simulink model "nms_3Dmodel_inv_wAnkleCPG"  (R2016b)
settings: Solver=ode3  StartTime=0.0  StopTime=tend  FixedStep=ts  RelTol=1e-3  EnableMultiTasking=on
InitFcn:
  | runScripts_inv;
values from neighbouring files (symbols this model uses):
  c = 0.05    [IID_nms_MechInit.m]    (also in nms_MechInit.m)
  c_jointstop = 0.3 / (pi/180)    (= 17.1887338539)    [IID_nms_MechInit.m]    (also in nms_MechInit.m)
  CPG_On = 1    [setCPGPar.m]    (also in setCPGPar_inv.m)
  CtrlPar_FP = [alpha0 alpha_cd alpha_cv]    [setCtrlPar.m]
  CtrlPar_FP_R = [R_hipR0 R_hipR_cd R_hipR_cv]    [setCtrlPar.m]
  CtrlPar_LL = l_clr    [setCtrlPar.m]
  CtrlPar_St = [StPreStim St_M1 St_M2 St_M3 St_M4 St_M5 St_M11]    [setCtrlPar.m]
  CtrlPar_St_R = [R_StPreStim R_St_M1 R_St_M3 R_St_M4]    [setCtrlPar.m]
  CtrlPar_Sw = [SwPreStim SwPhasePari SwPhaseParii SwCtrlPar_H SwCtrlPar_A      SwCtrlPar_Ki SwCtrlPar_Kii SwCtrlPar_Kiii SwCtrlPar_StP]    [setCtrlPar.m]
  CtrlPar_Sw_R = [R_SwPreStim R_Sw_M6]    [setCtrlPar.m]
  CtrlPar_theta0 = parBlCtrl(1)      *1*pi/180    [setCtrlPar.m]
  CtrlPar_Tr = [Tr_St_sup Tr_Sw]    [setCtrlPar.m]
  CtrlPar_Tr_R = [R_Tr_St_sup R_Tr_Sw]    [setCtrlPar.m]
  eref = 0.04    [IID_nms_MechInit.m]    (also in nms_MechInit.m)
  FmaxBFSH = 350    [nms_MechInit.m]
  FmaxGAS = 1500    [IID_nms_MechInit.m]    (also in nms_MechInit.m)
  FmaxGLU = 1500    [IID_nms_MechInit.m]    (also in nms_MechInit.m)
  FmaxHAB = 3000    [nms_MechInit.m]
  FmaxHAD = 4500    [nms_MechInit.m]
  FmaxHAM = 3000    [IID_nms_MechInit.m]    (also in nms_MechInit.m)
  FmaxHFL = 2000    [IID_nms_MechInit.m]    (also in nms_MechInit.m)
  FmaxRF = 1200    [nms_MechInit.m]
  FmaxSOL = 4000    [IID_nms_MechInit.m]    (also in nms_MechInit.m)
  FmaxTA = 800    [IID_nms_MechInit.m]    (also in nms_MechInit.m)
  FmaxVAS = 6000    [IID_nms_MechInit.m]    (also in nms_MechInit.m)
  init_a_tgt = 70*pi/180    (= 1.2217304764)    [setInitPar.m]
  init_a_tgtR = 90*pi/180    (= 1.57079632679)    [setInitPar.m]
  K = 5    [IID_nms_MechInit.m]    (also in nms_MechInit.m)
  leg_l = [D12_T D12_S]    [nms_MechInit.m]
  LongDelay = 0.020    (= 0.02)    [IID_setCtrlPar.m]    (also in nms_MechInit.m = 0.01)
  LongLoopDelay = 0.030    (= 0.03)    [nms_MechInit.m]
  loptBFSH = 0.12    [nms_MechInit.m]
  loptGAS = 0.05    [IID_nms_MechInit.m]    (also in nms_MechInit.m)
  loptGLU = 0.11    [IID_nms_MechInit.m]    (also in nms_MechInit.m)
  loptHAB = 0.09    [nms_MechInit.m]
  loptHAD = 0.10    (= 0.1)    [nms_MechInit.m]
  loptHAM = 0.10    (= 0.1)    [IID_nms_MechInit.m]    (also in nms_MechInit.m)
  loptHFL = 0.11    [IID_nms_MechInit.m]    (also in nms_MechInit.m)
  loptRF = 0.08    [nms_MechInit.m]
  loptSOL = 0.04    [IID_nms_MechInit.m]    (also in nms_MechInit.m)
  loptTA = 0.06    [IID_nms_MechInit.m]    (also in nms_MechInit.m)
  loptVAS = 0.08    [IID_nms_MechInit.m]    (also in nms_MechInit.m)
  lslackBFSH = 0.10    (= 0.1)    [nms_MechInit.m]
  lslackGAS = 0.40    (= 0.4)    [IID_nms_MechInit.m]    (also in nms_MechInit.m)
  lslackGLU = 0.13    [IID_nms_MechInit.m]    (also in nms_MechInit.m)
  lslackHAB = 0.07    [nms_MechInit.m]
  lslackHAD = 0.18    [nms_MechInit.m]
  lslackHAM = 0.31    [IID_nms_MechInit.m]    (also in nms_MechInit.m)
  lslackHFL = 0.10    (= 0.1)    [IID_nms_MechInit.m]    (also in nms_MechInit.m)
  lslackRF = 0.35    [nms_MechInit.m]
  lslackSOL = 0.26    [IID_nms_MechInit.m]    (also in nms_MechInit.m)
  lslackTA = 0.24    [IID_nms_MechInit.m]    (also in nms_MechInit.m)
  lslackVAS = 0.23    [IID_nms_MechInit.m]    (also in nms_MechInit.m)
  massBFSH = 2    [nms_MechInit.m]
  massGAS = 0.45    [IID_nms_MechInit.m]    (also in nms_MechInit.m)
  massGLU = 1.4    [IID_nms_MechInit.m]    (also in nms_MechInit.m)
  massHAB = 1.145    [nms_MechInit.m]
  massHAD = 1.91    [nms_MechInit.m]
  massHAM = 1.82    [IID_nms_MechInit.m]    (also in nms_MechInit.m)
  massHFL = 1.87    [IID_nms_MechInit.m]    (also in nms_MechInit.m)
  massRF = 1    [nms_MechInit.m]
  massSOL = 1.36    [IID_nms_MechInit.m]    (also in nms_MechInit.m)
  massTA = 0.29    [IID_nms_MechInit.m]    (also in nms_MechInit.m)
  massVAS = 2.91    [IID_nms_MechInit.m]    (also in nms_MechInit.m)
  MidDelay = 0.010    (= 0.01)    [IID_setCtrlPar.m]    (also in nms_MechInit.m = 0.005)
  N = 1.5    [IID_nms_MechInit.m]    (also in cmaes_parfor.m = size(x,1); nms_MechInit.m)
  phi12_LowLimit = 70*pi/180    (= 1.2217304764)    [IID_nms_MechInit.m]    (also in nms_MechInit.m)
  phi12_UpLimit = 130*pi/180    (= 2.26892802759)    [IID_nms_MechInit.m]    (also in nms_MechInit.m)
  phi23_UpLimit = 175*pi/180    (= 3.05432619099)    [IID_nms_MechInit.m]    (also in nms_MechInit.m)
  phi34_UpLimit = 230*pi/180    (= 4.01425727959)    [IID_nms_MechInit.m]    (also in nms_MechInit.m)
  phi34R_LowLimit = -15*pi/180    (= -0.261799387799)    [nms_MechInit.m]
  phi34R_UpLimit = 50*pi/180    (= 0.872664625997)    [nms_MechInit.m]
  phimaxGASa = 110*pi/180    (= 1.91986217719)    [IID_nms_MechInit.m]    (also in nms_MechInit.m = 1.74532925199)
  phimaxGASk = 140*pi/180    (= 2.44346095279)    [IID_nms_MechInit.m]    (also in nms_MechInit.m)
  phimaxRFk = 165*pi/180    (= 2.87979326579)    [nms_MechInit.m]
  phimaxSOL = 110*pi/180    (= 1.91986217719)    [IID_nms_MechInit.m]    (also in nms_MechInit.m = 1.74532925199)
  phimaxTA = 80*pi/180    (= 1.3962634016)    [IID_nms_MechInit.m]    (also in nms_MechInit.m)
  phimaxVAS = 165*pi/180    (= 2.87979326579)    [IID_nms_MechInit.m]    (also in nms_MechInit.m)
  phirefBFSH = 160*pi/180    (= 2.79252680319)    [nms_MechInit.m]
  phirefGASa = 80*pi/180    (= 1.3962634016)    [IID_nms_MechInit.m]    (also in nms_MechInit.m)
  phirefGASk = 165*pi/180    (= 2.87979326579)    [IID_nms_MechInit.m]    (also in nms_MechInit.m)
  phirefGLU = 150*pi/180    (= 2.61799387799)    [IID_nms_MechInit.m]    (also in nms_MechInit.m = 2.09439510239)
  phirefHAB = 10*pi/180    (= 0.174532925199)    [nms_MechInit.m]
  phirefHAD = 15*pi/180    (= 0.261799387799)    [nms_MechInit.m]
  phirefHAMh = 155*pi/180    (= 2.70526034059)    [IID_nms_MechInit.m]    (also in nms_MechInit.m = 2.61799387799)
  phirefHAMk = 180*pi/180    (= 3.14159265359)    [IID_nms_MechInit.m]    (also in nms_MechInit.m)
  phirefHFL = 180*pi/180    (= 3.14159265359)    [IID_nms_MechInit.m]    (also in nms_MechInit.m = 2.79252680319)
  phirefRFh = 170*pi/180    (= 2.96705972839)    [nms_MechInit.m]
  phirefRFk = 125*pi/180    (= 2.18166156499)    [nms_MechInit.m]
  phirefSOL = 80*pi/180    (= 1.3962634016)    [IID_nms_MechInit.m]    (also in nms_MechInit.m = 1.57079632679)
  phirefTA = 110*pi/180    (= 1.91986217719)    [IID_nms_MechInit.m]    (also in nms_MechInit.m)
  phirefVAS = 125*pi/180    (= 2.18166156499)    [IID_nms_MechInit.m]    (also in nms_MechInit.m = 2.09439510239)
  phiScaleGASa = acos(rGASamin/rGASamax)/(phiminGASa-phimaxGASa)    [nms_MechInit.m]
  phiScaleGASk = acos(rGASkmin/rGASkmax)/(phiminGASk-phimaxGASk)    [nms_MechInit.m]
  phiScaleRFk = acos(rRFkmin/rRFkmax)/(phiminRFk-phimaxRFk)    [nms_MechInit.m]
  phiScaleSOL = acos(rSOLmin/rSOLmax)/(phiminSOL-phimaxSOL)    [nms_MechInit.m]
  phiScaleTA = acos(rTAmin/rTAmax)/(phiminTA-phimaxTA)    [nms_MechInit.m]
  phiScaleVAS = acos(rVASmin/rVASmax)/(phiminVAS-phimaxVAS)    [nms_MechInit.m]
  rBFSH = 0.04    [nms_MechInit.m]
  rGASamax = 0.06    [nms_MechInit.m]
  rGASkmax = 0.05    [nms_MechInit.m]
  rGLU = 0.10    (= 0.1)    [IID_nms_MechInit.m]    (also in nms_MechInit.m = 0.08)
  rHAB = 0.06    [nms_MechInit.m]
  rHAD = 0.03    [nms_MechInit.m]
  rHAMh = 0.08    [IID_nms_MechInit.m]    (also in nms_MechInit.m)
  rHAMk = 0.05    [IID_nms_MechInit.m]    (also in nms_MechInit.m)
  rHFL = 0.10    (= 0.1)    [IID_nms_MechInit.m]    (also in nms_MechInit.m = 0.08)
  rhoBFSH = 0.7    [nms_MechInit.m]
  rhoGASa = 0.7    [IID_nms_MechInit.m]    (also in nms_MechInit.m)
  rhoGASk = 0.7    [IID_nms_MechInit.m]    (also in nms_MechInit.m)
  rhoGLU = 0.5    [IID_nms_MechInit.m]    (also in nms_MechInit.m)
  rhoHAB = 0.7    [nms_MechInit.m]
  rhoHAD = 1    [nms_MechInit.m]
  rhoHAMh = 0.7    [IID_nms_MechInit.m]    (also in nms_MechInit.m = 0.5)
  rhoHAMk = 0.7    [IID_nms_MechInit.m]    (also in nms_MechInit.m = 0.5)
  rhoHFL = 0.5    [IID_nms_MechInit.m]    (also in nms_MechInit.m)
  rhoRFh = 0.3    [nms_MechInit.m]
  rhoRFk = 0.5    [nms_MechInit.m]
  rhoSOL = 0.5    [IID_nms_MechInit.m]    (also in nms_MechInit.m)
  rhoTA = 0.7    [IID_nms_MechInit.m]    (also in nms_MechInit.m)
  ... (+55 more)
libraries: simulink_extras x30, nmc x30, simulink x22, NMCCPG_Library x13, powerlib_meascontrol x5
(part 3 of 12)

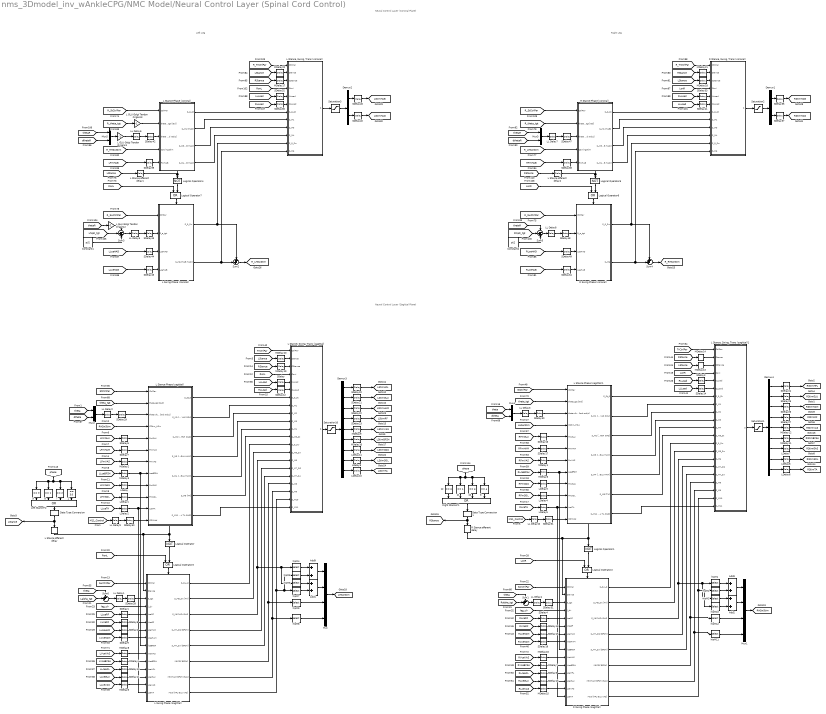
== system nms_3Dmodel_inv_wAnkleCPG/NMC Model/Neural Control Layer (Spinal Cord Control) ==
  note: Left Leg
  note: Right Leg
  note: Neural Control Layer
      | (Coronal Plane)
  note: Neural Control Layer
      | (Sagittal Plane)
  " 2" : simulink/Logic and Bit Operations/Compare To Constant  relop===  const=3.0  OutDataTypeStr=boolean
  " 3" : simulink/Logic and Bit Operations/Compare To Constant  relop===  const=4  OutDataTypeStr=boolean
  10 : simulink/Logic and Bit Operations/Compare To Constant  relop===  const=3  OutDataTypeStr=boolean
  11 : simulink/Logic and Bit Operations/Compare To Constant  relop===  const=1  OutDataTypeStr=boolean
  12 : simulink/Logic and Bit Operations/Compare To Constant  relop===  const=0  OutDataTypeStr=boolean
  7 : simulink/Logic and Bit Operations/Compare To Constant  relop===  const=2  OutDataTypeStr=boolean
  8 : simulink/Logic and Bit Operations/Compare To Constant  relop===  const=1  OutDataTypeStr=boolean
  9 : simulink/Logic and Bit Operations/Compare To Constant  relop===  const=0  OutDataTypeStr=boolean
  Add{1..3,9} (4 alike) : Sum  Inputs=2
  Constant1 : Constant  Value=pi/2
  Constant2 : Constant  Value=pi/2
  Data Type Conversion : DataTypeConversion
  Data Type Conversion1 : DataTypeConversion
  Demux1 : Demux  Outputs=2
  Demux2 : Demux  Outputs=2
  Demux3 : Demux  Outputs=9
  Demux4 : Demux  Outputs=9
  L GLU Golgi Tendon Organs1 : Gain  Gain=-1
  L GLU Golgi Tendon Organs2 : Gain  Gain=-1
  L GLU Golgi Tendon Organs3 : Gain  Gain=-1
  L Stance afferent delay : TransportDelay  DelayTime=MidDelay
  L Stance afferent delay1 : TransportDelay  DelayTime=MidDelay
  L Stance afferent delay2 : TransportDelay  DelayTime=MidDelay
  L Stance Phase (coronal) : Subsystem  TreatAsAtomicUnit=on
  L Stance Phase (sagittal) : Subsystem  TreatAsAtomicUnit=on
  L Stance Phase (sagittal)1 : Subsystem  TreatAsAtomicUnit=on
  "L Stance, Swing, Trans (coronal)" : Subsystem  TreatAsAtomicUnit=on
  "L Stance, Swing, Trans (sagittal)" : Subsystem
  "L Stance, Swing, Trans (sagittal)1" : Subsystem
  L Swing Phase (coronal) : Subsystem  TreatAsAtomicUnit=on
  L Swing Phase (sagittal) : Subsystem  TreatAsAtomicUnit=on
  LDelay{,1,3..4} (4 alike) : TransportDelay  DelayTime=LongDelay
  LDelay10 : TransportDelay  DelayTime=LongDelay  InitialOutput=St_PreSTA
  LDelay11 : TransportDelay  DelayTime=LongDelay  InitialOutput=St_PreSGAS
  LDelay2 : TransportDelay  DelayTime=LongDelay  InitialOutput=1
  LDelay5 : TransportDelay  DelayTime=LongDelay  InitialOutput=1
  LDelay6 : TransportDelay  DelayTime=LongDelay  InitialOutput=Sw_PreSTA
  LDelay7 : TransportDelay  DelayTime=LongDelay  InitialOutput=Sw_PreSGAS
  LDelay8 : TransportDelay  DelayTime=LongDelay  InitialOutput=Sw_PreSSOL
  LDelay9 : TransportDelay  DelayTime=LongDelay  InitialOutput=St_PreSSOL
  LL Delay1 : TransportDelay  DelayTime=LongLoopDelay/2  InitialOutput=init_a_tgt
  LL Delay{2..3,6..7,9..10} (6 alike) : TransportDelay  DelayTime=LongLoopDelay/2
  LL Delay4 : TransportDelay  DelayTime=LongLoopDelay/2  InitialOutput=init_a_tgt
  LL Delay5 : TransportDelay  DelayTime=LongLoopDelay/2  InitialOutput=init_a_tgtR
  LL Delay8 : TransportDelay  DelayTime=LongLoopDelay/2  InitialOutput=init_a_tgtR
  Left Stance?2 : Logic  Operator=OR  Inputs=4  AllPortsSameDT=off
  Logical Operator{,1,4..5} (4 alike) : Logic  Operator=NOT  AllPortsSameDT=off  OutDataTypeStr=boolean
  Logical Operator{2..3,6..7} (4 alike) : Logic  Operator=OR  AllPortsSameDT=off  OutDataTypeStr=boolean
  MDelay{1..2,4,7..8,13..14,16..22} (14 alike) : TransportDelay  DelayTime=MidDelay
  MDelay10 : TransportDelay  DelayTime=MidDelay  InitialOutput=St_PreSBFSH
  MDelay11 : TransportDelay  DelayTime=MidDelay  InitialOutput=Sw_PreSBFSH
  MDelay12 : TransportDelay  DelayTime=MidDelay  InitialOutput=Sw_PreSVAS
  MDelay{3,5..6,15} (4 alike) : TransportDelay  DelayTime=MidDelay  InitialOutput=1
  MDelay9 : TransportDelay  DelayTime=MidDelay  InitialOutput=St_PreSVAS
  Mux : Mux
  Mux1 : Mux
  Mux{2..5} (4 alike) : Mux  Inputs=2
  R Stance afferent delay : TransportDelay  DelayTime=MidDelay
  R Stance Phase (coronal) : Subsystem  TreatAsAtomicUnit=on
  "R Stance, Swing, Trans (coronal)" : Subsystem  TreatAsAtomicUnit=on
  R Swing Phase (coronal) : Subsystem  TreatAsAtomicUnit=on
  R Swing Phase (sagittal) : Subsystem  TreatAsAtomicUnit=on
  Right Stance?1 : Logic  Operator=OR  Inputs=4  AllPortsSameDT=off
  SDelay{,3,6..9,12,14,16..19,29..30,32..33,36,38..39,41..42,47,50..51} (24 alike) : TransportDelay  DelayTime=ShortDelay
  SDelay{1..2,4..5,10..11,13,15,34,44..45,49} (12 alike) : TransportDelay  DelayTime=ShortDelay  InitialOutput=1
  SDelay20 : TransportDelay  DelayTime=ShortDelay  InitialOutput=St_PreSHFL
  SDelay21 : TransportDelay  DelayTime=ShortDelay  InitialOutput=St_PreSGLU
  SDelay22 : TransportDelay  DelayTime=ShortDelay  InitialOutput=St_PreSHAM
  SDelay23 : TransportDelay  DelayTime=ShortDelay  InitialOutput=St_PreSRF
  SDelay24 : TransportDelay  DelayTime=ShortDelay  InitialOutput=Sw_PreSHFL
  SDelay25 : TransportDelay  DelayTime=ShortDelay  InitialOutput=Sw_PreSGLU
  SDelay26 : TransportDelay  DelayTime=ShortDelay  InitialOutput=Sw_PreSHAM
  SDelay27 : TransportDelay  DelayTime=ShortDelay  InitialOutput=Sw_PreSRF
  SDelay28 : TransportDelay  DelayTime=ShortDelay  InitialOutput=init_a_tgt
  SDelay31 : TransportDelay  DelayTime=ShortDelay  InitialOutput=init_a_tgt
  SDelay35 : TransportDelay  DelayTime=ShortDelay  InitialOutput=Sw_PreS_HAB
  SDelay37 : TransportDelay  DelayTime=ShortDelay  InitialOutput=Sw_PreS_HAD
  SDelay40 : TransportDelay  DelayTime=ShortDelay  InitialOutput=St_PreS_HAD
  SDelay43 : TransportDelay  DelayTime=ShortDelay  InitialOutput=init_a_tgtR
  SDelay46 : TransportDelay  DelayTime=ShortDelay  InitialOutput=St_PreS_HAB
  SDelay48 : TransportDelay  DelayTime=ShortDelay  InitialOutput=init_a_tgtR
  Saturation{1..3,10} (4 alike) : Saturate  UpperLimit=1  LowerLimit=0.01  ZeroCross=off
  Sum1 : Sum  Inputs=-+|
  Sum2 : Sum  Inputs=++|
  Sum3 : Sum  Inputs=--+
  Sum4 : Sum  Inputs=++|
  Sum5 : Sum  Inputs=--+
  Sum6 : Sum  Inputs=-+|
  hipM{1,4,9,12} (4 alike) : Selector  InputPortWidth=2  IndexOptions=Index vector (dialog)  Indices=1  OutputSizes=1
  hipM10 : Selector  InputPortWidth=3  IndexOptions=Index vector (dialog)  Indices=2  OutputSizes=1
  hipM{2,5,8,11} (4 alike) : Selector  InputPortWidth=3  IndexOptions=Index vector (dialog)  Indices=1  OutputSizes=1
  hipM3 : Selector  InputPortWidth=2  IndexOptions=Index vector (dialog)  Indices=2  OutputSizes=1
  hipM6 : Selector  InputPortWidth=2  IndexOptions=Index vector (dialog)  Indices=2  OutputSizes=1
  hipM7 : Selector  InputPortWidth=3  IndexOptions=Index vector (dialog)  Indices=2  OutputSizes=1
  tag scope: LHSwStim=global, LStance=global, LStimBFSH=global, LStimGAS=global, LStimGLU=global, LStimHAB=global, LStimHAD=global, LStimHAM=global, LStimHFL=global, LStimRF=global, LStimSOL=global, LStimTA=global, LStimVAS=global, RHSwStim=global, RStance=global, RStimBFSH=global, RStimGAS=global, RStimGLU=global, RStimHAB=global, RStimHAD=global, RStimHAM=global, RStimHFL=global, RStimRF=global, RStimSOL=global, RStimTA=global, RStimVAS=global, R_LHSwStim=global, R_RHSwStim=global
  wires:
  SDelay51/1 -> L Stance Phase (sagittal)1/12(COMVel)
  LL Delay10/1 -> SDelay51/1
  SDelay50/1 -> L Stance Phase (sagittal)/12(COMVel)
  LL Delay9/1 -> SDelay50/1
  [M11_Control] -> LL Delay10/1
  [M11_Control] -> LL Delay9/1
  L Stance Phase (sagittal)1/7(S_M11 [SOL TA GAS]) -> "L Stance, Swing, Trans (sagittal)1"/21(S_M11)
  L Stance Phase (sagittal)/7(S_M11 [SOL TA GAS]) -> "L Stance, Swing, Trans (sagittal)"/21(S_M11)
  SDelay37/1 -> [RStimHAD]
  SDelay35/1 -> [RStimHAB]
  SDelay39/1 -> L Stance Phase (coronal)/5(FmHAB)
  [LFmHAB] -> SDelay39/1
  L Stance Phase (coronal)/2(S_M1 [HAB]) -> "L Stance, Swing, Trans (coronal)"/8(S_M1)
  [dthetaR] -> Mux5/2
  [thetaR] -> Mux5/1
  L GLU Golgi Tendon Organs2/1 -> Sum3/1
  [thetaR] -> L GLU Golgi Tendon Organs2/1
  [LhipR_tgt] -> Sum3/2
  "L Stance, Swing, Trans (coronal)"/1(S) -> Saturation3/1
  SDelay40/1 -> [LStimHAD]
  SDelay46/1 -> [LStimHAB]
  MDelay17/1 -> "L Stance, Swing, Trans (coronal)"/3(CStance)
  MDelay22/1 -> "L Stance, Swing, Trans (coronal)"/2(Stance)
  SDelay45/1 -> L Swing Phase (coronal)/4(LceHAB)
  SDelay44/1 -> L Swing Phase (coronal)/3(LceHAD)
  Sum3/1 -> LL Delay5/1
  SDelay43/1 -> L Swing Phase (coronal)/2(R_a_tgt)
  LL Delay5/1 -> SDelay43/1
  L GLU Golgi Tendon Organs1/1 -> LL Delay6/1
  SDelay42/1 -> L Stance Phase (coronal)/3(theta dtheta [rad rad/s])
  LL Delay6/1 -> SDelay42/1
  Constant1/1 -> Sum3/3
  [LLceHAB] -> SDelay45/1
  [LLceHAD] -> SDelay44/1
  L Swing Phase (coronal)/1(S_0_Sw) -> Sum2/1, "L Stance, Swing, Trans (coronal)"/11(S_0_Sw)
  L Stance Phase (coronal)/4(S_M4 [HAB HAD]) -> "L Stance, Swing, Trans (coronal)"/10(S_M4)
  L Stance Phase (coronal)/3(S_M3 [HAB HAD]) -> "L Stance, Swing, Trans (coronal)"/9(S_M3)
  L Stance Phase (coronal)/1(S_0_St) -> "L Stance, Swing, Trans (coronal)"/7(S_0_St)
  SDelay32/1 -> "L Stance, Swing, Trans (coronal)"/5(ILLoad)
  Sum2/1 -> [R_LHSwStim]
  L Swing Phase (coronal)/2(S_M6 [HAB HAD]) -> "L Stance, Swing, Trans (coronal)"/12(S_M6), Sum2/2
  Mux5/1 -> L GLU Golgi Tendon Organs1/1
  [R_theta_tgt] -> L GLU Golgi Tendon Organs3/1
  [LLLoad] -> SDelay32/1
  Demux2/1 -> SDelay46/1
  Demux2/2 -> SDelay40/1
  Saturation3/1 -> Demux2/1
  SDelay36/1 -> "L Stance, Swing, Trans (coronal)"/6(CLLoad)
  [RLLoad] -> SDelay36/1
  [RStance] -> MDelay17/1
  [LStance] -> MDelay22/1
  [RonL] -> "L Stance, Swing, Trans (coronal)"/4(ConI)
  [R_TrCtrlPar] -> "L Stance, Swing, Trans (coronal)"/1(CtrlPar)
  [R_SwCtrlPar] -> L Swing Phase (coronal)/1(CtrlPar)
  [R_RHSwStim] -> L Stance Phase (coronal)/4(CSwingStim)
  [R_StCtrlPar] -> L Stance Phase (coronal)/1(CtrlPar)
  L GLU Golgi Tendon Organs3/1 -> L Stance Phase (coronal)/2(theta_tgt [rad])
  L Stance afferent delay1/1 -> L Stance Phase (coronal)/Enable, Logical Operator4/1
  [LStance] -> L Stance afferent delay1/1
  [RonL] -> Logical Operator7/1
  Logical Operator7/1 -> L Swing Phase (coronal)/Enable
  Logical Operator4/1 -> Logical Operator7/2
  SDelay38/1 -> R Stance Phase (coronal)/5(FmHAB)
  [RFmHAB] -> SDelay38/1
  R Stance Phase (coronal)/2(S_M1 [HAB]) -> "R Stance, Swing, Trans (coronal)"/8(S_M1)
  [dthetaR] -> Mux3/2
  [thetaR] -> Mux3/1
  "R Stance, Swing, Trans (coronal)"/1(S) -> Saturation2/1
  MDelay18/1 -> "R Stance, Swing, Trans (coronal)"/3(CStance)
  [LStance] -> MDelay18/1
  [RStance] -> MDelay21/1
  MDelay21/1 -> "R Stance, Swing, Trans (coronal)"/2(Stance)
  SDelay34/1 -> R Swing Phase (coronal)/4(LceHAB)
  SDelay49/1 -> R Swing Phase (coronal)/3(LceHAD)
  Sum5/1 -> LL Delay8/1
  SDelay48/1 -> R Swing Phase (coronal)/2(R_a_tgt)
  LL Delay8/1 -> SDelay48/1
  Mux3/1 -> LL Delay7/1
  SDelay47/1 -> R Stance Phase (coronal)/3(theta dtheta [rad rad/s])
  LL Delay7/1 -> SDelay47/1
  [thetaR] -> Sum5/1
  Constant2/1 -> Sum5/3
  [RhipR_tgt] -> Sum5/2
  [RLceHAB] -> SDelay34/1
  [RLceHAD] -> SDelay49/1
  R Swing Phase (coronal)/1(S_0_Sw) -> "R Stance, Swing, Trans (coronal)"/11(S_0_Sw), Sum4/1
  R Stance Phase (coronal)/4(S_M4 [HAB HAD]) -> "R Stance, Swing, Trans (coronal)"/10(S_M4)
  R Stance Phase (coronal)/3(S_M3 [HAB HAD]) -> "R Stance, Swing, Trans (coronal)"/9(S_M3)
  R Stance Phase (coronal)/1(S_0_St) -> "R Stance, Swing, Trans (coronal)"/7(S_0_St)
  SDelay33/1 -> "R Stance, Swing, Trans (coronal)"/5(ILLoad)
  Sum4/1 -> [R_RHSwStim]
  R Swing Phase (coronal)/2(S_M6) -> "R Stance, Swing, Trans (coronal)"/12(S_M6), Sum4/2
  [R_theta_tgt] -> R Stance Phase (coronal)/2(theta_tgt [rad])
  [RLLoad] -> SDelay33/1
  Demux1/1 -> SDelay35/1
  Demux1/2 -> SDelay37/1
  Saturation2/1 -> Demux1/1
  SDelay41/1 -> "R Stance, Swing, Trans (coronal)"/6(CLLoad)
  [LLLoad] -> SDelay41/1
  [LonR] -> "R Stance, Swing, Trans (coronal)"/4(ConI)
  [R_TrCtrlPar] -> "R Stance, Swing, Trans (coronal)"/1(CtrlPar)
  [R_SwCtrlPar] -> R Swing Phase (coronal)/1(CtrlPar)
  [R_LHSwStim] -> R Stance Phase (coronal)/4(CSwingStim)
  [R_StCtrlPar] -> R Stance Phase (coronal)/1(CtrlPar)
  L Stance afferent delay2/1 -> R Stance Phase (coronal)/Enable, Logical Operator5/1
  [RStance] -> L Stance afferent delay2/1
  [LonR] -> Logical Operator6/1
  Logical Operator6/1 -> R Swing Phase (coronal)/Enable
  Logical Operator5/1 -> Logical Operator6/2
  MDelay16/1 -> R Swing Phase (sagittal)/10(VceVAS)
  [RVceVAS] -> MDelay16/1
  MDelay8/1 -> L Swing Phase (sagittal)/10(VceVAS)
  [LVceVAS] -> MDelay8/1
  SDelay31/1 -> R Swing Phase (sagittal)/3(a_tgt)
  Sum1/1 -> LL Delay4/1
  LL Delay4/1 -> SDelay31/1
  hipM11/1 -> Mux1/4
  hipM12/1 -> Mux1/3
  Add2/1 -> Mux1/2
  hipM10/1 -> Add2/2
  hipM3/1 -> Add2/1
  Add3/1 -> Mux1/1
  hipM2/1 -> Add3/2
  hipM1/1 -> Add3/1
  Mux1/1 -> [RHSwStim]
  R Swing Phase (sagittal)/8(M10 [HFL GLU VAS]) -> hipM10/1, hipM2/1, "L Stance, Swing, Trans (sagittal)1"/20(S_M10)
  R Swing Phase (sagittal)/7(M9 [HAM BFSH GAS]) -> hipM11/1, "L Stance, Swing, Trans (sagittal)1"/19(S_M9)
  R Swing Phase (sagittal)/6(M8 [RF BFSH]) -> hipM12/1, "L Stance, Swing, Trans (sagittal)1"/18(S_M8)
  R Swing Phase (sagittal)/5(S_M7_Sw [BFSH]) -> "L Stance, Swing, Trans (sagittal)1"/17(S_M7_Sw)
  R Swing Phase (sagittal)/4(S_M7_DS [BFSH]) -> "L Stance, Swing, Trans (sagittal)1"/16(S_M7_DS)
  R Swing Phase (sagittal)/3(S_M6 [HFL GLU]) -> hipM1/1, hipM3/1, "L Stance, Swing, Trans (sagittal)1"/15(S_M6)
  R Swing Phase (sagittal)/2(S_M5_Sw [TA]) -> "L Stance, Swing, Trans (sagittal)1"/14(S_M5_Sw)
  R Swing Phase (sagittal)/1(S_Sw_0) -> "L Stance, Swing, Trans (sagittal)1"/13(S_0_Sw)
  "L Stance, Swing, Trans (sagittal)1"/1(S) -> Saturation1/1
  hipM8/1 -> Mux/4
  hipM9/1 -> Mux/3
  Add1/1 -> Mux/2
  hipM7/1 -> Add1/2
  hipM6/1 -> Add1/1
  Add9/1 -> Mux/1
  hipM5/1 -> Add9/2
  hipM4/1 -> Add9/1
  Mux/1 -> [LHSwStim]
  L Swing Phase (sagittal)/8(M10 [HFL GLU VAS]) -> hipM7/1, hipM5/1, "L Stance, Swing, Trans (sagittal)"/20(S_M10)
  L Swing Phase (sagittal)/7(M9 [HAM BFSH GAS]) -> hipM8/1, "L Stance, Swing, Trans (sagittal)"/19(S_M9)
  L Swing Phase (sagittal)/6(M8 [RF BFSH]) -> hipM9/1, "L Stance, Swing, Trans (sagittal)"/18(S_M8)
  L Swing Phase (sagittal)/5(S_M7_Sw [BFSH]) -> "L Stance, Swing, Trans (sagittal)"/17(S_M7_Sw)
  L Swing Phase (sagittal)/4(S_M7_DS [BFSH]) -> "L Stance, Swing, Trans (sagittal)"/16(S_M7_DS)
  L Swing Phase (sagittal)/3(S_M6 [HFL GLU]) -> hipM4/1, hipM6/1, "L Stance, Swing, Trans (sagittal)"/15(S_M6)
  L Swing Phase (sagittal)/2(S_M5_Sw [TA]) -> "L Stance, Swing, Trans (sagittal)"/14(S_M5_Sw)
  L Stance Phase (sagittal)/5(S_M4 [HFL GLU HAM]) -> "L Stance, Swing, Trans (sagittal)"/11(S_M4)
  L Stance Phase (sagittal)1/5(S_M4 [HFL GLU HAM]) -> "L Stance, Swing, Trans (sagittal)1"/11(S_M4)
  SDelay30/1 -> L Stance Phase (sagittal)1/3(theta dtheta [rad rad/s])
  Mux4/1 -> LL Delay3/1
  LL Delay3/1 -> SDelay30/1
  SDelay29/1 -> L Stance Phase (sagittal)/3(theta dtheta [rad rad/s])
  Mux2/1 -> LL Delay2/1
  LL Delay2/1 -> SDelay29/1
  SDelay3/1 -> "L Stance, Swing, Trans (sagittal)1"/5(ILLoad)
  L Stance Phase (sagittal)1/4(S_M3 [HFL GLU HAM]) -> "L Stance, Swing, Trans (sagittal)1"/10(S_M3)
  L Stance Phase (sagittal)/4(S_M3 [HFL GLU HAM]) -> "L Stance, Swing, Trans (sagittal)"/10(S_M3)
  [theta_tgt] -> L Stance Phase (sagittal)1/2(theta_tgt [rad])
  [dtheta] -> Mux4/2
  [theta] -> Mux4/1
  SDelay/1 -> "L Stance, Swing, Trans (sagittal)"/5(ILLoad)
  [theta_tgt] -> L Stance Phase (sagittal)/2(theta_tgt [rad])
  [dtheta] -> Mux2/2
  [theta] -> Mux2/1
  L Stance Phase (sagittal)1/6(S_M5 [TA]) -> "L Stance, Swing, Trans (sagittal)1"/12(S_M5_St)
  L Stance Phase (sagittal)1/3(S_M2 [HAM VAS BFSH GAS]) -> "L Stance, Swing, Trans (sagittal)1"/9(S_M2)
  L Stance Phase (sagittal)1/2(S_M1 [GLU VAS SOL]) -> "L Stance, Swing, Trans (sagittal)1"/8(S_M1)
  L Stance Phase (sagittal)/6(S_M5 [TA]) -> "L Stance, Swing, Trans (sagittal)"/12(S_M5_St)
  L Stance Phase (sagittal)/3(S_M2 [HAM VAS BFSH GAS]) -> "L Stance, Swing, Trans (sagittal)"/9(S_M2)
  L Stance Phase (sagittal)/2(S_M1 [GLU VAS SOL]) -> "L Stance, Swing, Trans (sagittal)"/8(S_M1)
  L Stance Phase (sagittal)1/1(S_St_0) -> "L Stance, Swing, Trans (sagittal)1"/7(S_0_St)
  L Swing Phase (sagittal)/1(S_Sw_0) -> "L Stance, Swing, Trans (sagittal)"/13(S_0_Sw)
  L Stance Phase (sagittal)/1(S_St_0) -> "L Stance, Swing, Trans (sagittal)"/7(S_0_St)
  SDelay28/1 -> L Swing Phase (sagittal)/3(a_tgt)
  Sum6/1 -> LL Delay1/1
  LL Delay1/1 -> SDelay28/1
  [RLceVAS] -> MDelay15/1
  [RLceGLU] -> SDelay13/1
  [RLceHFL] -> SDelay5/1
  [LLceVAS] -> MDelay5/1
  [LLceGLU] -> SDelay11/1
  [LLceHFL] -> SDelay10/1
  MDelay13/1 -> "L Stance, Swing, Trans (sagittal)1"/3(CStance)
  MDelay14/1 -> "L Stance, Swing, Trans (sagittal)1"/2(Stance)
  MDelay19/1 -> "L Stance, Swing, Trans (sagittal)"/3(CStance)
  MDelay20/1 -> "L Stance, Swing, Trans (sagittal)"/2(Stance)
  [theta] -> Sum1/1
  [Ralpha_tgt] -> Sum1/2
  [theta] -> Sum6/1
  [Lalpha_tgt] -> Sum6/2
  LDelay6/1 -> [RStimTA]
  LDelay8/1 -> [RStimSOL]
  LDelay7/1 -> [RStimGAS]
  MDelay11/1 -> [RStimBFSH]
  MDelay12/1 -> [RStimVAS]
  SDelay27/1 -> [RStimRF]
  SDelay26/1 -> [RStimHAM]
  SDelay25/1 -> [RStimGLU]
  SDelay24/1 -> [RStimHFL]
  Demux4/6 -> MDelay11/1
  Demux4/5 -> MDelay12/1
  Demux4/4 -> SDelay27/1
  Demux4/9 -> LDelay6/1
  Demux4/8 -> LDelay8/1
  Demux4/7 -> LDelay7/1
  Demux4/3 -> SDelay26/1
  Demux4/2 -> SDelay25/1
  Demux4/1 -> SDelay24/1
  LDelay10/1 -> [LStimTA]
  LDelay9/1 -> [LStimSOL]
  LDelay11/1 -> [LStimGAS]
  MDelay10/1 -> [LStimBFSH]
  MDelay9/1 -> [LStimVAS]
  SDelay23/1 -> [LStimRF]
  SDelay22/1 -> [LStimHAM]
  SDelay21/1 -> [LStimGLU]
  SDelay20/1 -> [LStimHFL]
  SDelay12/1 -> "L Stance, Swing, Trans (sagittal)"/6(CLLoad)
  [LStance] -> MDelay13/1
  [RStance] -> MDelay14/1
  [LonR] -> "L Stance, Swing, Trans (sagittal)1"/4(ConI)
  Saturation1/1 -> Demux4/1
  [LLLoad] -> SDelay14/1
  SDelay14/1 -> "L Stance, Swing, Trans (sagittal)1"/6(CLLoad)
  [TrCtrlPar] -> "L Stance, Swing, Trans (sagittal)1"/1(CtrlPar)
  MDelay15/1 -> R Swing Phase (sagittal)/14(LceVAS)
  SDelay13/1 -> R Swing Phase (sagittal)/13(LceGLU)
  SDelay5/1 -> R Swing Phase (sagittal)/12(LceHFL)
  MDelay7/1 -> R Swing Phase (sagittal)/11(VceBFSH)
  [RVceBFSH] -> MDelay7/1
  SDelay19/1 -> R Swing Phase (sagittal)/8(VceHAM)
  [RVceHAM] -> SDelay19/1
  SDelay18/1 -> R Swing Phase (sagittal)/6(VceRF)
  [RVceRF] -> SDelay18/1
  SDelay15/1 -> R Swing Phase (sagittal)/7(LceHAM)
  [RLceHAM] -> SDelay15/1
  SDelay4/1 -> R Swing Phase (sagittal)/5(LceRF)
  [RLceRF] -> SDelay4/1
  [leg_clr] -> R Swing Phase (sagittal)/4(l_clr)
  [LonR] -> Logical Operator2/1
  Logical Operator2/1 -> R Swing Phase (sagittal)/Enable
  Logical Operator1/1 -> Logical Operator2/2
  R Stance afferent delay/1 -> L Stance Phase (sagittal)1/Enable, Logical Operator1/1, R Swing Phase (sagittal)/2(Stance)
  [SwCtrlPar] -> R Swing Phase (sagittal)/1(CtrlPar)
  LDelay5/1 -> L Stance Phase (sagittal)1/11(LceTA), R Swing Phase (sagittal)/15(LceTA)
  [RLceTA] -> LDelay5/1
  LDelay4/1 -> L Stance Phase (sagittal)1/10(FmSOL)
  [RFmSOL] -> LDelay4/1
  LDelay3/1 -> L Stance Phase (sagittal)1/9(FmGAS)
  [RFmGAS] -> LDelay3/1
  MDelay6/1 -> L Stance Phase (sagittal)1/8(LceBFSH), R Swing Phase (sagittal)/9(lceBFSH)
  [RLceBFSH] -> MDelay6/1
  MDelay1/1 -> L Stance Phase (sagittal)1/7(FmVAS)
  [RFmVAS] -> MDelay1/1
  SDelay17/1 -> L Stance Phase (sagittal)1/6(FmHAM)
  [RFmHAM] -> SDelay17/1
  SDelay16/1 -> L Stance Phase (sagittal)1/5(FmGLU)
  [RFmGLU] -> SDelay16/1
  [LHSwStim] -> L Stance Phase (sagittal)1/4(CStim_HSw)
  [RLLoad] -> SDelay3/1
  [StCtrlPar] -> L Stance Phase (sagittal)1/1(CtrlPar)
  Right Stance?1/1 -> Data Type Conversion1/1
  [RStance] -> MDelay19/1
  [LStance] -> MDelay20/1
  [RonL] -> "L Stance, Swing, Trans (sagittal)"/4(ConI)
  "L Stance, Swing, Trans (sagittal)"/1(S) -> Saturation10/1
  Demux3/6 -> MDelay10/1
  Demux3/5 -> MDelay9/1
  Demux3/4 -> SDelay23/1
  Demux3/9 -> LDelay10/1
  Demux3/8 -> LDelay9/1
  Demux3/7 -> LDelay11/1
  Saturation10/1 -> Demux3/1
  Demux3/3 -> SDelay22/1
  Demux3/2 -> SDelay21/1
  Demux3/1 -> SDelay20/1
  [RLLoad] -> SDelay12/1
  [TrCtrlPar] -> "L Stance, Swing, Trans (sagittal)"/1(CtrlPar)
  MDelay5/1 -> L Swing Phase (sagittal)/14(LceVAS)
  SDelay11/1 -> L Swing Phase (sagittal)/13(LceGLU)
  SDelay10/1 -> L Swing Phase (sagittal)/12(LceHFL)
  MDelay4/1 -> L Swing Phase (sagittal)/11(VceBFSH)
  [LVceBFSH] -> MDelay4/1
  SDelay9/1 -> L Swing Phase (sagittal)/8(VceHAM)
  [LVceHAM] -> SDelay9/1
  SDelay8/1 -> L Swing Phase (sagittal)/6(VceRF)
  [LVceRF] -> SDelay8/1
  SDelay2/1 -> L Swing Phase (sagittal)/7(LceHAM)
  [LLceHAM] -> SDelay2/1
  SDelay1/1 -> L Swing Phase (sagittal)/5(LceRF)
  [LLceRF] -> SDelay1/1
  [leg_clr] -> L Swing Phase (sagittal)/4(l_clr)
  [RonL] -> Logical Operator3/1
  Logical Operator3/1 -> L Swing Phase (sagittal)/Enable
  Logical Operator/1 -> Logical Operator3/2
  L Stance afferent delay/1 -> L Swing Phase (sagittal)/2(Stance), Logical Operator/1, L Stance Phase (sagittal)/Enable
  [SwCtrlPar] -> L Swing Phase (sagittal)/1(CtrlPar)
  LDelay2/1 -> L Stance Phase (sagittal)/11(LceTA), L Swing Phase (sagittal)/15(LceTA)
  [LLceTA] -> LDelay2/1
  LDelay1/1 -> L Stance Phase (sagittal)/10(FmSOL)
  [LFmSOL] -> LDelay1/1
  LDelay/1 -> L Stance Phase (sagittal)/9(FmGAS)
  [LFmGAS] -> LDelay/1
  MDelay3/1 -> L Stance Phase (sagittal)/8(LceBFSH), L Swing Phase (sagittal)/9(lceBFSH)
  [LLceBFSH] -> MDelay3/1
  MDelay2/1 -> L Stance Phase (sagittal)/7(FmVAS)
  [LFmVAS] -> MDelay2/1
  SDelay7/1 -> L Stance Phase (sagittal)/6(FmHAM)
  [LFmHAM] -> SDelay7/1
  SDelay6/1 -> L Stance Phase (sagittal)/5(FmGLU)
  [LFmGLU] -> SDelay6/1
  [RHSwStim] -> L Stance Phase (sagittal)/4(CStim_HSw)
  [StCtrlPar] -> L Stance Phase (sagittal)/1(CtrlPar)
  Left Stance?2/1 -> Data Type Conversion/1
  [LLLoad] -> SDelay/1
  9/1 -> Left Stance?2/1
  8/1 -> Left Stance?2/2
  7/1 -> Left Stance?2/3
  " 2"/1 -> Left Stance?2/4
  [phase] -> " 2"/1, 7/1, 9/1, 8/1
  12/1 -> Right Stance?1/1
  11/1 -> Right Stance?1/2
  10/1 -> Right Stance?1/3
  " 3"/1 -> Right Stance?1/4
  [phase] -> " 3"/1, 10/1, 12/1, 11/1
  Data Type Conversion/1 -> [LStance], L Stance afferent delay/1
  Data Type Conversion1/1 -> [RStance], R Stance afferent delay/1

== system nms_3Dmodel_inv_wAnkleCPG/NMC Model/etc ==
  note: Control Parameters
  Clock : Clock
  Constant10 : Constant  Value=CtrlPar_Tr
  Constant11 : Constant  Value=CtrlPar_Tr_R
  Constant12 : Constant  Value=CtrlPar_theta0
  Constant2 : Constant  Value=CtrlPar_LL
  Constant3 : Constant  Value=CtrlPar_St_R
  Constant5 : Constant  Value=CtrlPar_St
  Constant6 : Constant  Value=CtrlPar_FP
  Constant7 : Constant  Value=CtrlPar_FP_R
  Constant8 : Constant  Value=CtrlPar_Sw_R
  Constant9 : Constant  Value=CtrlPar_Sw
  To Current Workspace2 : ToWorkspace  VariableName=simout_tEnd  SaveFormat=Structure  SampleTime=-1
      settings: MaxDataPoints=1
  tag scope: FPCtrlPar=global, LLCtrlPar=global, R_FPCtrlPar=global, R_StCtrlPar=global, R_SwCtrlPar=global, R_TrCtrlPar=global, StCtrlPar=global, SwCtrlPar=global, TrCtrlPar=global, theta0=global
  wires:
  Clock/1 -> To Current Workspace2/1
  Constant10/1 -> [TrCtrlPar]
  Constant11/1 -> [R_TrCtrlPar]
  Constant8/1 -> [R_SwCtrlPar]
  Constant7/1 -> [R_FPCtrlPar]
  Constant3/1 -> [R_StCtrlPar]
  Constant12/1 -> [theta0]
  Constant5/1 -> [StCtrlPar]
  Constant2/1 -> [LLCtrlPar]
  Constant9/1 -> [SwCtrlPar]
  Constant6/1 -> [FPCtrlPar]

== system nms_3Dmodel_inv_wAnkleCPG/NMC Model/CPG/CPG Output ==
  CPG_on_Left : Subsystem
  Current Phase Left : Subsystem
  Shape estimator left : Subsystem
  tag scope: front_v_est=global
  wires:
  CPG_on_Left/1(CPG_On) -> Shape estimator left/Enable
  Shape estimator left/1(Shape) -> [front_v_est]
  Current Phase Left/1(cur_phase) -> Shape estimator left/1(Cur_phase)

== system nms_3Dmodel_inv_wAnkleCPG/NMC Model/CPG/Etc ==
  Detect_change : NMCCPG_Library/Detect_change
  Logical Operator1 : Logic  Inputs=4  AllPortsSameDT=off  OutDataTypeStr=boolean
  Memory : Memory
  Product : Product
  Sample and Hold{,1..3} (4 alike) : powerlib_meascontrol/Additional Components/Sample and Hold  ic=0  Ts=0
  tag scope: Saved_kept=global, Switch=global
  wires:
  Sample and Hold3/1 -> Logical Operator1/4
  Sample and Hold2/1 -> Logical Operator1/3
  [Saved_Ph3] -> Sample and Hold2/2, Sample and Hold2/1
  [Saved_Ph4] -> Sample and Hold3/1, Sample and Hold3/2
  [Saved_Ph1] -> Sample and Hold/2, Sample and Hold/1
  [Saved_Ph2] -> Sample and Hold1/1, Sample and Hold1/2
  Sample and Hold1/1 -> Logical Operator1/2
  Sample and Hold/1 -> Logical Operator1/1
  Logical Operator1/1 -> [Saved_kept]
  Detect_change/1 -> Product/1
  Product/1 -> Memory/1
  [phase] -> Product/2, Detect_change/1
  Memory/1 -> [Switch]

== system nms_3Dmodel_inv_wAnkleCPG/NMC Model/CPG/Learning center ==
  note: Phases
  Phase 1 : Subsystem  mask{Phase='1'}
      mask prompts: Phase "Which Phase?"
      mask init:
      | blk = gcb;
      | set_param([gcb '/rec_sig'],'Value',Phase);
      | 
      | set_param([gcb '/save_sig'],'GotoTag',['Saved_Ph',Phase]);
      | 
      | set_param([gcb '/SaveToWorkspace/data_store_shape'],'DataStoreName',['Shape_Ph',Phase]);
      | set_param([gcb '/SaveToWorkspace/data_store_freq'],'DataStoreName',['Freq_Ph',Phase]);
  Phase 2 : Subsystem  mask{Phase='2'}
      mask prompts: Phase "Which Phase?"
      mask init: same as nms_3Dmodel_inv_wAnkleCPG/NMC Model/CPG/Learning center/Phase 1
  Phase 3 : Subsystem  mask{Phase='3'}
      mask prompts: Phase "Which Phase?"
      mask init: same as nms_3Dmodel_inv_wAnkleCPG/NMC Model/CPG/Learning center/Phase 1
  Phase 4 : Subsystem  mask{Phase='4'}
      mask prompts: Phase "Which Phase?"
      mask init: same as nms_3Dmodel_inv_wAnkleCPG/NMC Model/CPG/Learning center/Phase 1

== system nms_3Dmodel_inv_wAnkleCPG/NMC Model/Higher Control Layer (Supra Spinal Control)/Double Support ==
  LStance : Inport
  RStance : Inport  Port=2
  Lalpha_tgt : Inport  Port=3
  Lphi34 : Inport  Port=4
  Lphi23 : Inport  Port=5
  LHip_tgt : Inport  Port=6
  Lphi34R : Inport  Port=7
  Ralpha_tgt : Inport  Port=8
  Rphi34 : Inport  Port=9
  Rphi23 : Inport  Port=10
  RHip_tgt : Inport  Port=11
  Rphi34R : Inport  Port=12
  Abs{,1..3} (4 alike) : Abs  ZeroCross=off
  Lalpha' : Fcn  Expr=u(1) - u(2)/2
  Logical Operator1 : Logic  Operator=NOR  AllPortsSameDT=off  OutDataTypeStr=boolean
  Logical Operator2 : Logic  Operator=NOT  AllPortsSameDT=off
  Logical Operator3 : Logic  AllPortsSameDT=off
  Logical Operator4 : Logic  AllPortsSameDT=off
  Logical Operator5 : Logic  AllPortsSameDT=off
  Mux1 : Mux  Inputs=2
  Mux5 : Mux  Inputs=2
  Ralpha' : Fcn  Expr=u(1) - u(2)/2
  Relational Operator : RelationalOperator  Operator=>  ZeroCross=off  RndMeth=Nearest
  Sum{1,3,5,7} (4 alike) : Sum  Inputs=-+|
  Sum2 : Sum  Inputs=++|
  Sum4 : Sum  Inputs=++|
  RonL : Outport
  Flight : Outport  Port=2
  LonR : Outport  Port=3
  wires:
  Logical Operator3/1 -> Logical Operator4/1, Logical Operator5/1
  Relational Operator/1 -> Logical Operator4/2, Logical Operator2/1
  Logical Operator5/1 -> LonR/1
  Logical Operator2/1 -> Logical Operator5/2
  Logical Operator4/1 -> RonL/1
  Sum4/1 -> Relational Operator/2
  Abs3/1 -> Sum4/1
  Abs/1 -> Sum4/2
  Sum3/1 -> Abs3/1
  Rphi34R/1 -> Sum3/2
  RHip_tgt/1 -> Sum3/1
  Sum2/1 -> Relational Operator/1
  Abs1/1 -> Sum2/2
  Abs2/1 -> Sum2/1
  Sum1/1 -> Abs2/1
  Lphi34R/1 -> Sum1/2
  LHip_tgt/1 -> Sum1/1
  Logical Operator1/1 -> Flight/1
  Rphi23/1 -> Mux1/2
  Rphi34/1 -> Mux1/1
  Ralpha_tgt/1 -> Sum5/1
  Lphi23/1 -> Mux5/2
  Lphi34/1 -> Mux5/1
  Lalpha_tgt/1 -> Sum7/1
  RStance/1 -> Logical Operator1/2, Logical Operator3/2
  LStance/1 -> Logical Operator1/1, Logical Operator3/1
  Sum7/1 -> Abs1/1
  Sum5/1 -> Abs/1
  Mux1/1 -> Ralpha'/1
  Ralpha'/1 -> Sum5/2
  Mux5/1 -> Lalpha'/1
  Lalpha'/1 -> Sum7/2  "Lalpha"

== system nms_3Dmodel_inv_wAnkleCPG/NMC Model/Muscle Actuation Layer/F GAS ==
  note: Excitation Contraction Coupling
  note: GAS Muscle-Tendon Dynamics
  STIM : Inport
  lmtc [m] : Inport  Port=2
  1 : Product  Inputs=**  SaturateOnIntegerOverflow=on  InputSameDT=on  OutDataTypeStr=Inherit: Same as first input
  1/lslack : Gain  Gain=1/lslackGAS  SaturateOnIntegerOverflow=on  OutDataTypeStr=Inherit: Same as input  ParamDataTypeStr=Inherit: Same as input
  2 : Product  Inputs=***  SaturateOnIntegerOverflow=on  InputSameDT=on  OutDataTypeStr=Inherit: Same as first input
  BE force-length relation : Subsystem
  CE force-length relation : Subsystem
  CE inverse force-velocity relation : Subsystem
  Constant : Constant  Value=lslackGAS
  ECC TransferFcn : simulink_extras/Additional Linear/Transfer Fcn (with initial outputs)  N=[1]  D="[tau  1]"  Y0=preA  U0=0
      settings: AttributesFormatString=pre-activation: %<Y0>
  Fmax : Gain  Gain=FmaxGAS  SaturateOnIntegerOverflow=on  OutDataTypeStr=Inherit: Same as input  ParamDataTypeStr=Inherit: Same as input
  Fmax1 : Gain  Gain=FmaxGAS  SaturateOnIntegerOverflow=on  OutDataTypeStr=Inherit: Same as input  ParamDataTypeStr=Inherit: Same as input
  Fv = Fse / (A*Fce) : Product  Inputs=*/  SaturateOnIntegerOverflow=on  InputSameDT=on  OutDataTypeStr=Inherit: Same as first input
  Integrator : Integrator  InitialConditionSource=external  LowerSaturationLimit=0.05  ZeroCross=off
  PE force-length relation : Subsystem
  SE force-length relation : Subsystem
  Sum : Sum  Inputs=|+-  SaturateOnIntegerOverflow=on  InputSameDT=on  OutDataTypeStr=Inherit: Same as first input
  Sum2 : Sum  Inputs=|-+  SaturateOnIntegerOverflow=on  InputSameDT=on  OutDataTypeStr=Inherit: Same as first input
  Sum3 : Sum  SaturateOnIntegerOverflow=on  InputSameDT=on  OutDataTypeStr=Inherit: Same as first input
  Sum4 : Sum  SaturateOnIntegerOverflow=on  InputSameDT=on  OutDataTypeStr=Inherit: Same as first input
  lce/lopt : Gain  Gain=1/loptGAS  SaturateOnIntegerOverflow=on  OutDataTypeStr=Inherit: Same as input  ParamDataTypeStr=Inherit: Same as input
  vmax*lopt : Gain  Gain=vmaxGAS*loptGAS  SaturateOnIntegerOverflow=on  OutDataTypeStr=Inherit: Same as input  ParamDataTypeStr=Inherit: Same as input
  Fmtc : Outport  InitialOutput=0
  Lce : Outport  Port=2  InitialOutput=0
  Vce : Outport  Port=3  InitialOutput=0
  A : Outport  Port=4  InitialOutput=0
  Fac : Outport  Port=5  InitialOutput=0
  wires:
  Fmax1/1 -> Fac/1
  2/1 -> Fmax1/1
  ECC TransferFcn/1 -> 1/2, A/1, 2/2  "A"
  CE force-length relation/1(fce [Fmax]) -> 1/1, 2/1  "fl"
  Fv = Fse / (A*Fce)/1 -> CE inverse force-velocity relation/1(Fv[Fmax]), 2/3  "fv"
  STIM/1 -> ECC TransferFcn/1
  CE inverse force-velocity relation/1(v[vmax]) -> vmax*lopt/1
  Sum3/1 -> Fv = Fse / (A*Fce)/2
  BE force-length relation/1(fbe [Fmax]) -> Sum4/2
  1/1 -> Sum3/2
  PE force-length relation/1(fpe [Fmax]) -> Sum3/1
  Sum4/1 -> Fv = Fse / (A*Fce)/1
  Constant/1 -> Sum2/1
  Sum2/1 -> Integrator/2
  SE force-length relation/1(fse [Fmax]) -> Sum4/1, Fmax/1
  1/lslack/1 -> SE force-length relation/1(lse [lslack])
  Fmax/1 -> Fmtc/1  "Fmtc"
  lmtc [m]/1 -> Sum/1, Sum2/2  "lmtc"
  vmax*lopt/1 -> Vce/1, Integrator/1  "vce"
  lce/lopt/1 -> PE force-length relation/1(lce [lopt]), BE force-length relation/1(lce [lopt]), CE force-length relation/1(lce [lopt])
  Sum/1 -> 1/lslack/1  "lse"
  Integrator/1 -> Lce/1, lce/lopt/1, Sum/2  "lce"

== system nms_3Dmodel_inv_wAnkleCPG/NMC Model/Muscle Actuation Layer/L Ankle Joint Limits ==
  note: Ankle Joint Limits
  phi [rad] : Inport
  dphi [rad/s] : Inport  Port=2
  Gain1 : Gain  Gain=c_jointstop
  Gain2 : Gain  Gain=-1
  Gain3 : Gain  Gain=c_jointstop
  Gain4 : Gain  Gain=1/w_max_jointstop
  Limit Ankle Range : simulink/Logic and Bit Operations/Interval Test  IntervalClosedRight=on  uplimit=phi12_UpLimit + 40*pi/180  IntervalClosedLeft=on  lowlimit=phi12_LowLimit - 40*pi/180  OutDataTypeStr=boolean
  Logical Operator3 : Logic  Operator=NOT  AllPortsSameDT=off  OutDataTypeStr=boolean
  Mux1 : Mux  Inputs=2
  Mux3 : Mux  Inputs=2
  Overextension Torque : Fcn  Expr="- u(1)  *  (1-u(2)) * (u(2)<1) * (u(1)>0)"
  Overflexion Torque : Fcn  Expr="- u(1)  *  (1-u(2)) * (u(2)<1) * (u(1)<0)"
  Stop Simulation1 : Stop
  Sum : Sum  Inputs=|+-
  Sum1 : Sum  Inputs=|+-
  Sum2 : Sum
  overextension angle : Constant  Value=phi12_UpLimit
  overflexion angle : Constant  Value=phi12_LowLimit
  M_stop [Nm] : Outport
  wires:
  Logical Operator3/1 -> Stop Simulation1/1
  Limit Ankle Range/1 -> Logical Operator3/1
  Overextension Torque/1 -> Sum2/1
  Overflexion Torque/1 -> Sum2/2
  Gain2/1 -> Mux3/2
  Sum2/1 -> M_stop [Nm]/1
  Mux1/1 -> Overflexion Torque/1
  overflexion angle/1 -> Sum1/2
  Sum1/1 -> Gain1/1
  Gain1/1 -> Mux1/1
  Gain4/1 -> Mux1/2, Gain2/1
  Sum/1 -> Gain3/1
  phi [rad]/1 -> Limit Ankle Range/1, Sum1/1, Sum/1
  overextension angle/1 -> Sum/2
  dphi [rad/s]/1 -> Gain4/1
  Gain3/1 -> Mux3/1
  Mux3/1 -> Overextension Torque/1

== system nms_3Dmodel_inv_wAnkleCPG/NMC Model/Muscle Actuation Layer/L BFSH ==
  note: Excitation Contraction Coupling
  note: BFSH Muscle-Tendon Dynamics
  STIM : Inport
  lmtc [m] : Inport  Port=2
  1 : Product  Inputs=**  SaturateOnIntegerOverflow=on  InputSameDT=on  OutDataTypeStr=Inherit: Same as first input
  1/lslack : Gain  Gain=1/lslackBFSH  SaturateOnIntegerOverflow=on  OutDataTypeStr=Inherit: Same as input  ParamDataTypeStr=Inherit: Same as input
  2 : Product  Inputs=***  SaturateOnIntegerOverflow=on  InputSameDT=on  OutDataTypeStr=Inherit: Same as first input
  BE force-length relation : Subsystem
  CE force-length relation : Subsystem
  CE inverse force-velocity relation : Subsystem
  Constant : Constant  Value=lslackBFSH
  ECC TransferFcn : simulink_extras/Additional Linear/Transfer Fcn (with initial outputs)  N=[1]  D="[tau  1]"  Y0=preA  U0=0
      settings: AttributesFormatString=pre-activation: %<Y0>
  Fmax : Gain  Gain=FmaxBFSH  SaturateOnIntegerOverflow=on  OutDataTypeStr=Inherit: Same as input  ParamDataTypeStr=Inherit: Same as input
  Fmax1 : Gain  Gain=FmaxBFSH  SaturateOnIntegerOverflow=on  OutDataTypeStr=Inherit: Same as input  ParamDataTypeStr=Inherit: Same as input
  Fv = Fse / (A*Fce) : Product  Inputs=*/  SaturateOnIntegerOverflow=on  InputSameDT=on  OutDataTypeStr=Inherit: Same as first input
  Integrator : Integrator  InitialConditionSource=external  LowerSaturationLimit=0.05  ZeroCross=off
  PE force-length relation : Subsystem
  SE force-length relation : Subsystem
  Sum : Sum  Inputs=|+-  SaturateOnIntegerOverflow=on  InputSameDT=on  OutDataTypeStr=Inherit: Same as first input
  Sum2 : Sum  Inputs=|-+  SaturateOnIntegerOverflow=on  InputSameDT=on  OutDataTypeStr=Inherit: Same as first input
  Sum3 : Sum  SaturateOnIntegerOverflow=on  InputSameDT=on  OutDataTypeStr=Inherit: Same as first input
  Sum4 : Sum  SaturateOnIntegerOverflow=on  InputSameDT=on  OutDataTypeStr=Inherit: Same as first input
  lce/lopt : Gain  Gain=1/loptBFSH  SaturateOnIntegerOverflow=on  OutDataTypeStr=Inherit: Same as input  ParamDataTypeStr=Inherit: Same as input
  vmax*lopt : Gain  Gain=vmaxBFSH*loptBFSH  SaturateOnIntegerOverflow=on  OutDataTypeStr=Inherit: Same as input  ParamDataTypeStr=Inherit: Same as input
  Fmtc : Outport  InitialOutput=0
  Lce : Outport  Port=2  InitialOutput=0
  Vce : Outport  Port=3  InitialOutput=0
  A : Outport  Port=4  InitialOutput=0
  Fac : Outport  Port=5  InitialOutput=0
  wires:
  Fmax1/1 -> Fac/1
  2/1 -> Fmax1/1
  ECC TransferFcn/1 -> 1/2, A/1, 2/2  "A"
  CE force-length relation/1(fce [Fmax]) -> 1/1, 2/1  "fl"
  Fv = Fse / (A*Fce)/1 -> CE inverse force-velocity relation/1(Fv[Fmax]), 2/3  "fv"
  STIM/1 -> ECC TransferFcn/1
  CE inverse force-velocity relation/1(v[vmax]) -> vmax*lopt/1
  Sum3/1 -> Fv = Fse / (A*Fce)/2
  BE force-length relation/1(fbe [Fmax]) -> Sum4/2
  1/1 -> Sum3/2
  PE force-length relation/1(fpe [Fmax]) -> Sum3/1
  Sum4/1 -> Fv = Fse / (A*Fce)/1
  Constant/1 -> Sum2/1
  Sum2/1 -> Integrator/2
  SE force-length relation/1(fse [Fmax]) -> Sum4/1, Fmax/1
  1/lslack/1 -> SE force-length relation/1(lse [lslack])
  Fmax/1 -> Fmtc/1  "Fmtc"
  lmtc [m]/1 -> Sum/1, Sum2/2  "lmtc"
  vmax*lopt/1 -> Vce/1, Integrator/1  "vce"
  lce/lopt/1 -> PE force-length relation/1(lce [lopt]), BE force-length relation/1(lce [lopt]), CE force-length relation/1(lce [lopt])
  Sum/1 -> 1/lslack/1  "lse"
  Integrator/1 -> Lce/1, lce/lopt/1, Sum/2  "lce"

== system nms_3Dmodel_inv_wAnkleCPG/NMC Model/Muscle Actuation Layer/L BFSH Link ==
  note: BFSH Attachment
  phi23 [rad] : Inport
  Constant : Constant  Value=lslackBFSH+loptBFSH
  Constant1 : Constant  Value=rBFSH
  Constant2 : Constant  Value=phirefBFSH
  Gain4 : Gain  Gain=rhoBFSH
  Product : Product  RndMeth=Zero
  Sum2 : Sum  Inputs=|+-
  Sum5 : Sum  Inputs=|++
  lmtu [m] : Outport
  lever [m] : Outport  Port=2
  wires:
  Constant1/1 -> lever [m]/1, Product/2
  Sum2/1 -> Product/1
  Constant2/1 -> Sum2/2
  phi23 [rad]/1 -> Sum2/1
  Product/1 -> Gain4/1
  Gain4/1 -> Sum5/2
  Sum5/1 -> lmtu [m]/1
  Constant/1 -> Sum5/1

== system nms_3Dmodel_inv_wAnkleCPG/NMC Model/Muscle Actuation Layer/L GAS Link ==
  note: GAS Attachment
  phi23 [rad] : Inport
  phi12 [rad] : Inport  Port=2
  Constant1 : Constant  Value=phimaxGASk
  Constant2 : Constant  Value=phirefGASk
  Constant3 : Constant  Value=phimaxGASa
  Constant4 : Constant  Value=lslackGAS+loptGAS
  Constant5 : Constant  Value=phirefGASa
  Demux : Demux  Outputs=2
  Demux1 : Demux  Outputs=2
  Gain1 : Gain  Gain=rGASkmax
  Gain2 : Gain  Gain=rGASamax
  Gain3 : Gain  Gain=phiScaleGASa
  Gain5 : Gain  Gain=phiScaleGASk
  Gain6 : Gain  Gain=phiScaleGASk
  Gain7 : Gain  Gain=rhoGASk/phiScaleGASk
  Gain8 : Gain  Gain=phiScaleGASa
  Gain9 : Gain  Gain=rhoGASa/phiScaleGASa
  Mux : Mux  Inputs=2
  Mux1 : Mux  Inputs=2
  Sum1 : Sum  Inputs=-+
  Sum2 : Sum  Inputs=|+-
  Sum3 : Sum  Inputs=-+|
  Sum4 : Sum  Inputs=-+
  Sum5 : Sum  Inputs=++-
  Sum6 : Sum  Inputs=|+-
  Sum7 : Sum  Inputs=-+|
  length change term : Trigonometry
  length change term1 : Trigonometry
  offset correction term : Trigonometry
  offset correction term1 : Trigonometry
  variable lever term : Trigonometry  Operator=cos
  variable lever term1 : Trigonometry  Operator=cos
  lmtu [m] : Outport
  lever23 [m] : Outport  Port=2
  lever12 [m] : Outport  Port=3
  wires:
  Gain8/1 -> offset correction term1/1
  Gain3/1 -> length change term1/1, variable lever term1/1
  Gain2/1 -> Demux1/1
  Mux1/1 -> Gain2/1
  variable lever term1/1 -> Mux1/2
  Sum4/1 -> Mux1/1
  offset correction term1/1 -> Sum4/1
  length change term1/1 -> Sum4/2
  Constant5/1 -> Sum6/1
  Sum6/1 -> Gain8/1
  Constant3/1 -> Sum6/2, Sum7/1
  Sum7/1 -> Gain3/1
  phi12 [rad]/1 -> Sum7/2
  Gain6/1 -> offset correction term/1
  Gain5/1 -> length change term/1, variable lever term/1
  Gain1/1 -> Demux/1
  Mux/1 -> Gain1/1
  variable lever term/1 -> Mux/2
  Sum1/1 -> Mux/1
  offset correction term/1 -> Sum1/1
  length change term/1 -> Sum1/2
  Constant2/1 -> Sum2/1
  Sum2/1 -> Gain6/1
  Constant1/1 -> Sum2/2, Sum3/1
  Sum3/1 -> Gain5/1
  phi23 [rad]/1 -> Sum3/2
  Gain7/1 -> Sum5/1
  Demux/1 -> Gain7/1
  Demux/2 -> lever23 [m]/1
  Gain9/1 -> Sum5/3
  Demux1/1 -> Gain9/1
  Constant4/1 -> Sum5/2
  Demux1/2 -> lever12 [m]/1
  Sum5/1 -> lmtu [m]/1
